simulink model "DemonstratorSimscape"  (R2020b)
settings: Solver=ode113  StartTime=0.0  StopTime=t_stop*0+20  FixedStep=1e-4
values from neighbouring files (symbols this model uses):
  brkD = 0    [main.m]
  brkI = 1e4    (= 10000)    [main.m]
  brkP = 1e5    (= 100000)    [main.m]
  d_drm = 0.5*d_drum    [main.m]
  d_shm = 0.4*d_sheave    [main.m]
  DeltaCable0 = 0    [main.m]
  Droop_scaling = 0    [main.m]
  eta_sh = 0.015    [main.m]
  filt_NUM = ones(1,200)*0.005    [main.m]
  g = 9.80665    [main.m]
  Iw = 0.5*(W.i + M.in*GB.r^2)    [main.m]
  Kp_mul = 0.3    [main.m]
  Lc0 = abs((T.ph-L.height-P.d-L.z0)*0.001)    [main.m]
  Ls1 = ((T.ph-0.5*W.pd)/1000)    [main.m]
  Ls2 = ((0.5*(T.s2+P.d)-2*P.d)/1000)    [main.m]
  M = 50e3    (= 50000)    [calcGrav.m]
  phi0_drm = -90    [main.m]
  phi0_shm = -90    [main.m]
  r_sheave = P.d*0.5    [main.m]
  s = tf('s')    [calcGrav.m]
  tau_brk = 0.001    [main.m]
  tau_em = 60e-3    (= 0.06)    [calcGrav.m]    (also in main.m)
  tau_m = tau_w/GB.r    [main.m]
  Tmax = 400e3    (= 400000)    [main.m]
  Tn_mul = 10    [main.m]
  x_drm = 0.7*r_drum    [main.m]
  x_shm = 0.7*r_sheave    [main.m]
  z0 = 0    [calcGrav.m]    (also in main.m = L.z0-P.d*0.5-P.d-P.d-L.height-T.h1-T.h2-32)
undefined symbols (not defined in the file or in its folder): C, CA, Controller_sampleTime, DiscIntNeverNeededParam, GB, L, P, Part, T, VFD_acceleration_model_factor, VFD_Adapt_factor_lower_p1458, VFD_Adapt_factor_upper_p1459, VFD_Curr_limit_var_p0641, VFD_Current_limit_p0640, VFD_Id_setp_total_r1624, VFD_Iq, VFD_Kp_n_basic_p1460, VFD_M, VFD_M_accel_T_smooth_p1517, VFD_M_lim_var_fixS_src_p1551, VFD_M_max_lower_p1521, VFD_M_max_lower_scal_p1525, VFD_M_max_up_mot_scal_p1524, VFD_M_max_upper_p1520, VFD_n_act_T_smooth_p1442, VFD_n_ctr_Kp_n_up_scal_p1461, VFD_n_ctr_Tn_n_up_sca_p1463, VFD_n_ctrl_adapt_Kp_lower_p1456, VFD_n_ctrl_adapt_Kp_upper_p1457, VFD_n_ctrl_Adpt_sig_Kp_p1455, VFD_n_ctrl_Kp_scal_p1466, VFD_n_ctrl_n_lower_p1464, VFD_n_ctrl_n_upper_p1465, VFD_n_ctrl_Tn_n_lower_p1462, VFD_n_limit_neg_p1086, VFD_n_limit_pos_p1083, VFD_n_limit_setp_p1063, VFD_n_max_p1082, VFD_n_set_filt_1_T_p1416, VFD_P_max_gen_p1531, VFD_P_max_mot_p1530, VFD_PU_I_outp_max_r0289, VFD_RFG_ramp_down_time_p1121, VFD_RFG_ramp_up_time_p1120, VFD_RFG_t_RD_scal_p1139, VFD_RFG_t_RU_scal_p1138, VSD, W, X, Y, Z
libraries: sm_lib x248, nesl_utility x128, simulink x49, pid_lib x4, cstblocks x2, simulink_extras x2
(part 10 of 10)

== system DemonstratorSimscape/Transmission System/Roof Pulley Set/Sheave_04/Pulley rught red2/tags ==
  Rigid Transform1 : sm_lib/Frames and Transforms/Rigid Transform  TranslationMethod=Cartesian  TranslationStandardOffset=0  TranslationLengthUnit=mm  TranslationStandardAxis=+Z  TranslationCartesianOffset=[x_shm*cosd(phi0+120), x_shm*sind(phi0+120), s*d_shm]  TranslationROffset=0  TranslationROffsetUnits=m  TranslationZOffset=0  TranslationZOffsetUnits=m  TranslationThetaOffset=0  TranslationThetaOffsetUnits=deg  RotationMethod=None  RotationAngleUnits=deg  RotationStandardAxis=+Z  RotationAngle=0.0  RotationArbitraryAxis=[0 0 1]  FollAlignAxisA=+X  BaseAlignAxisA=+Y  FollAlignAxisB=+Y  BaseAlignAxisB=+Z  RotationSequenceAxes=FollowerAxes  RotationSequence=XYX  RotationSequenceAngles=[0 0 0]  RotationSequenceAnglesUnits=deg  RotationMatrix=[1 0 0; 0 1 0; 0 0 1]
  Rigid Transform2 : sm_lib/Frames and Transforms/Rigid Transform  TranslationMethod=Cartesian  TranslationStandardOffset=0  TranslationLengthUnit=mm  TranslationStandardAxis=+Z  TranslationCartesianOffset=[x_shm*cosd(phi0+0), x_shm*sind(phi0+0), s*d_shm]  TranslationROffset=0  TranslationROffsetUnits=m  TranslationZOffset=0  TranslationZOffsetUnits=m  TranslationThetaOffset=0  TranslationThetaOffsetUnits=deg  RotationMethod=None  RotationAngleUnits=deg  RotationStandardAxis=+Z  RotationAngle=0.0  RotationArbitraryAxis=[0 0 1]  FollAlignAxisA=+X  BaseAlignAxisA=+Y  FollAlignAxisB=+Y  BaseAlignAxisB=+Z  RotationSequenceAxes=FollowerAxes  RotationSequence=XYX  RotationSequenceAngles=[0 0 0]  RotationSequenceAnglesUnits=deg  RotationMatrix=[1 0 0; 0 1 0; 0 0 1]
  Rigid Transform3 : sm_lib/Frames and Transforms/Rigid Transform  TranslationMethod=Cartesian  TranslationStandardOffset=0  TranslationLengthUnit=mm  TranslationStandardAxis=+Z  TranslationCartesianOffset=[x_shm*cosd(phi0-120), x_shm*sind(phi0-120), s*d_shm]  TranslationROffset=0  TranslationROffsetUnits=m  TranslationZOffset=0  TranslationZOffsetUnits=m  TranslationThetaOffset=0  TranslationThetaOffsetUnits=deg  RotationMethod=None  RotationAngleUnits=deg  RotationStandardAxis=+Z  RotationAngle=0.0  RotationArbitraryAxis=[0 0 1]  FollAlignAxisA=+X  BaseAlignAxisA=+Y  FollAlignAxisB=+Y  BaseAlignAxisB=+Z  RotationSequenceAxes=FollowerAxes  RotationSequence=XYX  RotationSequenceAngles=[0 0 0]  RotationSequenceAnglesUnits=deg  RotationMatrix=[1 0 0; 0 1 0; 0 0 1]
  tag1 : sm_lib/Body Elements/Cylindrical Solid  GraphicAmbientColor=[0.15 0.15 0.15 1.0]  BasedOnType=Density  CenterOfMass=[0 0 0]  CenterOfMassUnits=m  GraphicDiffuseColor=c_shm  CylinderLength=d_shm  CylinderLengthUnits=mm  CylinderRadius=r_shm  CylinderRadiusUnits=mm  Density=0  DensityUnits=kg/m^3  DoExposeReferenceFrame=on  GraphicEmissiveColor=[0.0 0.0 0.0 1.0]  ExportEntireGeometry=off  SerializedFrames=<Frames/>  MarkerShape=Frame  MarkerSize=10  GraphicType=FromGeometry  InertiaType=CalculateFromGeometry  Mass=0  MassUnits=kg  MomentsOfInertia=[1 1 1]  MomentsOfInertiaUnits=kg*m^2  GraphicOpacity=1.0  ProductsOfInertia=[0 0 0]  ProductsOfInertiaUnits=kg*m^2  GraphicShininess=10  GraphicSpecularColor=[0.8 0.8 0.8]  GraphicVisPropType=SimpleVisualProperties
  tag2 : sm_lib/Body Elements/Cylindrical Solid  GraphicAmbientColor=[0.15 0.15 0.15 1.0]  BasedOnType=Density  CenterOfMass=[0 0 0]  CenterOfMassUnits=m  GraphicDiffuseColor=c_shm  CylinderLength=d_shm  CylinderLengthUnits=mm  CylinderRadius=r_shm  CylinderRadiusUnits=mm  Density=0  DensityUnits=kg/m^3  DoExposeReferenceFrame=on  GraphicEmissiveColor=[0.0 0.0 0.0 1.0]  ExportEntireGeometry=off  SerializedFrames=<Frames/>  MarkerShape=Frame  MarkerSize=10  GraphicType=FromGeometry  InertiaType=CalculateFromGeometry  Mass=0  MassUnits=kg  MomentsOfInertia=[1 1 1]  MomentsOfInertiaUnits=kg*m^2  GraphicOpacity=1.0  ProductsOfInertia=[0 0 0]  ProductsOfInertiaUnits=kg*m^2  GraphicShininess=10  GraphicSpecularColor=[0.8 0.8 0.8]  GraphicVisPropType=SimpleVisualProperties
  tag3 : sm_lib/Body Elements/Cylindrical Solid  GraphicAmbientColor=[0.15 0.15 0.15 1.0]  BasedOnType=Density  CenterOfMass=[0 0 0]  CenterOfMassUnits=m  GraphicDiffuseColor=c_shm  CylinderLength=d_shm  CylinderLengthUnits=mm  CylinderRadius=r_shm  CylinderRadiusUnits=mm  Density=0  DensityUnits=kg/m^3  DoExposeReferenceFrame=on  GraphicEmissiveColor=[0.0 0.0 0.0 1.0]  ExportEntireGeometry=off  SerializedFrames=<Frames/>  MarkerShape=Frame  MarkerSize=10  GraphicType=FromGeometry  InertiaType=CalculateFromGeometry  Mass=0  MassUnits=kg  MomentsOfInertia=[1 1 1]  MomentsOfInertiaUnits=kg*m^2  GraphicOpacity=1.0  ProductsOfInertia=[0 0 0]  ProductsOfInertiaUnits=kg*m^2  GraphicShininess=10  GraphicSpecularColor=[0.8 0.8 0.8]  GraphicVisPropType=SimpleVisualProperties
  Conn1 : PMIOPort  Side=Left
  connections:
  tag2/RConn1 -- Rigid Transform1/RConn1
  Conn1/RConn1 -- Rigid Transform2/LConn1 -- Rigid Transform1/LConn1 -- Rigid Transform3/LConn1
  Rigid Transform2/RConn1 -- tag1/RConn1
  Rigid Transform3/RConn1 -- tag3/RConn1

== system DemonstratorSimscape/Transmission System/Roof Pulley Set/Sheave_06/Sheave6/tags ==
  Rigid Transform1 : sm_lib/Frames and Transforms/Rigid Transform  TranslationMethod=Cartesian  TranslationStandardOffset=0  TranslationLengthUnit=mm  TranslationStandardAxis=+Z  TranslationCartesianOffset=[x_shm*cosd(phi0+120), x_shm*sind(phi0+120), s*d_shm]  TranslationROffset=0  TranslationROffsetUnits=m  TranslationZOffset=0  TranslationZOffsetUnits=m  TranslationThetaOffset=0  TranslationThetaOffsetUnits=deg  RotationMethod=None  RotationAngleUnits=deg  RotationStandardAxis=+Z  RotationAngle=0.0  RotationArbitraryAxis=[0 0 1]  FollAlignAxisA=+X  BaseAlignAxisA=+Y  FollAlignAxisB=+Y  BaseAlignAxisB=+Z  RotationSequenceAxes=FollowerAxes  RotationSequence=XYX  RotationSequenceAngles=[0 0 0]  RotationSequenceAnglesUnits=deg  RotationMatrix=[1 0 0; 0 1 0; 0 0 1]
  Rigid Transform2 : sm_lib/Frames and Transforms/Rigid Transform  TranslationMethod=Cartesian  TranslationStandardOffset=0  TranslationLengthUnit=mm  TranslationStandardAxis=+Z  TranslationCartesianOffset=[x_shm*cosd(phi0+0), x_shm*sind(phi0+0), s*d_shm]  TranslationROffset=0  TranslationROffsetUnits=m  TranslationZOffset=0  TranslationZOffsetUnits=m  TranslationThetaOffset=0  TranslationThetaOffsetUnits=deg  RotationMethod=None  RotationAngleUnits=deg  RotationStandardAxis=+Z  RotationAngle=0.0  RotationArbitraryAxis=[0 0 1]  FollAlignAxisA=+X  BaseAlignAxisA=+Y  FollAlignAxisB=+Y  BaseAlignAxisB=+Z  RotationSequenceAxes=FollowerAxes  RotationSequence=XYX  RotationSequenceAngles=[0 0 0]  RotationSequenceAnglesUnits=deg  RotationMatrix=[1 0 0; 0 1 0; 0 0 1]
  Rigid Transform3 : sm_lib/Frames and Transforms/Rigid Transform  TranslationMethod=Cartesian  TranslationStandardOffset=0  TranslationLengthUnit=mm  TranslationStandardAxis=+Z  TranslationCartesianOffset=[x_shm*cosd(phi0-120), x_shm*sind(phi0-120), s*d_shm]  TranslationROffset=0  TranslationROffsetUnits=m  TranslationZOffset=0  TranslationZOffsetUnits=m  TranslationThetaOffset=0  TranslationThetaOffsetUnits=deg  RotationMethod=None  RotationAngleUnits=deg  RotationStandardAxis=+Z  RotationAngle=0.0  RotationArbitraryAxis=[0 0 1]  FollAlignAxisA=+X  BaseAlignAxisA=+Y  FollAlignAxisB=+Y  BaseAlignAxisB=+Z  RotationSequenceAxes=FollowerAxes  RotationSequence=XYX  RotationSequenceAngles=[0 0 0]  RotationSequenceAnglesUnits=deg  RotationMatrix=[1 0 0; 0 1 0; 0 0 1]
  tag1 : sm_lib/Body Elements/Cylindrical Solid  GraphicAmbientColor=[0.15 0.15 0.15 1.0]  BasedOnType=Density  CenterOfMass=[0 0 0]  CenterOfMassUnits=m  GraphicDiffuseColor=c_shm  CylinderLength=d_shm  CylinderLengthUnits=mm  CylinderRadius=r_shm  CylinderRadiusUnits=mm  Density=0  DensityUnits=kg/m^3  DoExposeReferenceFrame=on  GraphicEmissiveColor=[0.0 0.0 0.0 1.0]  ExportEntireGeometry=off  SerializedFrames=<Frames/>  MarkerShape=Frame  MarkerSize=10  GraphicType=FromGeometry  InertiaType=CalculateFromGeometry  Mass=0  MassUnits=kg  MomentsOfInertia=[1 1 1]  MomentsOfInertiaUnits=kg*m^2  GraphicOpacity=1.0  ProductsOfInertia=[0 0 0]  ProductsOfInertiaUnits=kg*m^2  GraphicShininess=10  GraphicSpecularColor=[0.8 0.8 0.8]  GraphicVisPropType=SimpleVisualProperties
  tag2 : sm_lib/Body Elements/Cylindrical Solid  GraphicAmbientColor=[0.15 0.15 0.15 1.0]  BasedOnType=Density  CenterOfMass=[0 0 0]  CenterOfMassUnits=m  GraphicDiffuseColor=c_shm  CylinderLength=d_shm  CylinderLengthUnits=mm  CylinderRadius=r_shm  CylinderRadiusUnits=mm  Density=0  DensityUnits=kg/m^3  DoExposeReferenceFrame=on  GraphicEmissiveColor=[0.0 0.0 0.0 1.0]  ExportEntireGeometry=off  SerializedFrames=<Frames/>  MarkerShape=Frame  MarkerSize=10  GraphicType=FromGeometry  InertiaType=CalculateFromGeometry  Mass=0  MassUnits=kg  MomentsOfInertia=[1 1 1]  MomentsOfInertiaUnits=kg*m^2  GraphicOpacity=1.0  ProductsOfInertia=[0 0 0]  ProductsOfInertiaUnits=kg*m^2  GraphicShininess=10  GraphicSpecularColor=[0.8 0.8 0.8]  GraphicVisPropType=SimpleVisualProperties
  tag3 : sm_lib/Body Elements/Cylindrical Solid  GraphicAmbientColor=[0.15 0.15 0.15 1.0]  BasedOnType=Density  CenterOfMass=[0 0 0]  CenterOfMassUnits=m  GraphicDiffuseColor=c_shm  CylinderLength=d_shm  CylinderLengthUnits=mm  CylinderRadius=r_shm  CylinderRadiusUnits=mm  Density=0  DensityUnits=kg/m^3  DoExposeReferenceFrame=on  GraphicEmissiveColor=[0.0 0.0 0.0 1.0]  ExportEntireGeometry=off  SerializedFrames=<Frames/>  MarkerShape=Frame  MarkerSize=10  GraphicType=FromGeometry  InertiaType=CalculateFromGeometry  Mass=0  MassUnits=kg  MomentsOfInertia=[1 1 1]  MomentsOfInertiaUnits=kg*m^2  GraphicOpacity=1.0  ProductsOfInertia=[0 0 0]  ProductsOfInertiaUnits=kg*m^2  GraphicShininess=10  GraphicSpecularColor=[0.8 0.8 0.8]  GraphicVisPropType=SimpleVisualProperties
  Conn1 : PMIOPort  Side=Left
  connections:
  tag2/RConn1 -- Rigid Transform1/RConn1
  Conn1/RConn1 -- Rigid Transform2/LConn1 -- Rigid Transform1/LConn1 -- Rigid Transform3/LConn1
  Rigid Transform2/RConn1 -- tag1/RConn1
  Rigid Transform3/RConn1 -- tag3/RConn1

== system DemonstratorSimscape/Transmission System/Roof Pulley Set/Sheave_07/Sheave7/tags ==
  Rigid Transform1 : sm_lib/Frames and Transforms/Rigid Transform  TranslationMethod=Cartesian  TranslationStandardOffset=0  TranslationLengthUnit=mm  TranslationStandardAxis=+Z  TranslationCartesianOffset=[x_shm*cosd(phi0+120), x_shm*sind(phi0+120), s*d_shm]  TranslationROffset=0  TranslationROffsetUnits=m  TranslationZOffset=0  TranslationZOffsetUnits=m  TranslationThetaOffset=0  TranslationThetaOffsetUnits=deg  RotationMethod=None  RotationAngleUnits=deg  RotationStandardAxis=+Z  RotationAngle=0.0  RotationArbitraryAxis=[0 0 1]  FollAlignAxisA=+X  BaseAlignAxisA=+Y  FollAlignAxisB=+Y  BaseAlignAxisB=+Z  RotationSequenceAxes=FollowerAxes  RotationSequence=XYX  RotationSequenceAngles=[0 0 0]  RotationSequenceAnglesUnits=deg  RotationMatrix=[1 0 0; 0 1 0; 0 0 1]
  Rigid Transform2 : sm_lib/Frames and Transforms/Rigid Transform  TranslationMethod=Cartesian  TranslationStandardOffset=0  TranslationLengthUnit=mm  TranslationStandardAxis=+Z  TranslationCartesianOffset=[x_shm*cosd(phi0+0), x_shm*sind(phi0+0), s*d_shm]  TranslationROffset=0  TranslationROffsetUnits=m  TranslationZOffset=0  TranslationZOffsetUnits=m  TranslationThetaOffset=0  TranslationThetaOffsetUnits=deg  RotationMethod=None  RotationAngleUnits=deg  RotationStandardAxis=+Z  RotationAngle=0.0  RotationArbitraryAxis=[0 0 1]  FollAlignAxisA=+X  BaseAlignAxisA=+Y  FollAlignAxisB=+Y  BaseAlignAxisB=+Z  RotationSequenceAxes=FollowerAxes  RotationSequence=XYX  RotationSequenceAngles=[0 0 0]  RotationSequenceAnglesUnits=deg  RotationMatrix=[1 0 0; 0 1 0; 0 0 1]
  Rigid Transform3 : sm_lib/Frames and Transforms/Rigid Transform  TranslationMethod=Cartesian  TranslationStandardOffset=0  TranslationLengthUnit=mm  TranslationStandardAxis=+Z  TranslationCartesianOffset=[x_shm*cosd(phi0-120), x_shm*sind(phi0-120), s*d_shm]  TranslationROffset=0  TranslationROffsetUnits=m  TranslationZOffset=0  TranslationZOffsetUnits=m  TranslationThetaOffset=0  TranslationThetaOffsetUnits=deg  RotationMethod=None  RotationAngleUnits=deg  RotationStandardAxis=+Z  RotationAngle=0.0  RotationArbitraryAxis=[0 0 1]  FollAlignAxisA=+X  BaseAlignAxisA=+Y  FollAlignAxisB=+Y  BaseAlignAxisB=+Z  RotationSequenceAxes=FollowerAxes  RotationSequence=XYX  RotationSequenceAngles=[0 0 0]  RotationSequenceAnglesUnits=deg  RotationMatrix=[1 0 0; 0 1 0; 0 0 1]
  tag1 : sm_lib/Body Elements/Cylindrical Solid  GraphicAmbientColor=[0.15 0.15 0.15 1.0]  BasedOnType=Density  CenterOfMass=[0 0 0]  CenterOfMassUnits=m  GraphicDiffuseColor=c_shm  CylinderLength=d_shm  CylinderLengthUnits=mm  CylinderRadius=r_shm  CylinderRadiusUnits=mm  Density=0  DensityUnits=kg/m^3  DoExposeReferenceFrame=on  GraphicEmissiveColor=[0.0 0.0 0.0 1.0]  ExportEntireGeometry=off  SerializedFrames=<Frames/>  MarkerShape=Frame  MarkerSize=10  GraphicType=FromGeometry  InertiaType=CalculateFromGeometry  Mass=0  MassUnits=kg  MomentsOfInertia=[1 1 1]  MomentsOfInertiaUnits=kg*m^2  GraphicOpacity=1.0  ProductsOfInertia=[0 0 0]  ProductsOfInertiaUnits=kg*m^2  GraphicShininess=10  GraphicSpecularColor=[0.8 0.8 0.8]  GraphicVisPropType=SimpleVisualProperties
  tag2 : sm_lib/Body Elements/Cylindrical Solid  GraphicAmbientColor=[0.15 0.15 0.15 1.0]  BasedOnType=Density  CenterOfMass=[0 0 0]  CenterOfMassUnits=m  GraphicDiffuseColor=c_shm  CylinderLength=d_shm  CylinderLengthUnits=mm  CylinderRadius=r_shm  CylinderRadiusUnits=mm  Density=0  DensityUnits=kg/m^3  DoExposeReferenceFrame=on  GraphicEmissiveColor=[0.0 0.0 0.0 1.0]  ExportEntireGeometry=off  SerializedFrames=<Frames/>  MarkerShape=Frame  MarkerSize=10  GraphicType=FromGeometry  InertiaType=CalculateFromGeometry  Mass=0  MassUnits=kg  MomentsOfInertia=[1 1 1]  MomentsOfInertiaUnits=kg*m^2  GraphicOpacity=1.0  ProductsOfInertia=[0 0 0]  ProductsOfInertiaUnits=kg*m^2  GraphicShininess=10  GraphicSpecularColor=[0.8 0.8 0.8]  GraphicVisPropType=SimpleVisualProperties
  tag3 : sm_lib/Body Elements/Cylindrical Solid  GraphicAmbientColor=[0.15 0.15 0.15 1.0]  BasedOnType=Density  CenterOfMass=[0 0 0]  CenterOfMassUnits=m  GraphicDiffuseColor=c_shm  CylinderLength=d_shm  CylinderLengthUnits=mm  CylinderRadius=r_shm  CylinderRadiusUnits=mm  Density=0  DensityUnits=kg/m^3  DoExposeReferenceFrame=on  GraphicEmissiveColor=[0.0 0.0 0.0 1.0]  ExportEntireGeometry=off  SerializedFrames=<Frames/>  MarkerShape=Frame  MarkerSize=10  GraphicType=FromGeometry  InertiaType=CalculateFromGeometry  Mass=0  MassUnits=kg  MomentsOfInertia=[1 1 1]  MomentsOfInertiaUnits=kg*m^2  GraphicOpacity=1.0  ProductsOfInertia=[0 0 0]  ProductsOfInertiaUnits=kg*m^2  GraphicShininess=10  GraphicSpecularColor=[0.8 0.8 0.8]  GraphicVisPropType=SimpleVisualProperties
  Conn1 : PMIOPort  Side=Left
  connections:
  tag2/RConn1 -- Rigid Transform1/RConn1
  Conn1/RConn1 -- Rigid Transform2/LConn1 -- Rigid Transform1/LConn1 -- Rigid Transform3/LConn1
  Rigid Transform2/RConn1 -- tag1/RConn1
  Rigid Transform3/RConn1 -- tag3/RConn1

== system DemonstratorSimscape/EM System/Drives/PLC and Drive Logic Rev3/VFD Control1/[6020] Speed control and generation of the torque limits /1st order LPF ==
  Signal : Inport
  Time Constant : Inport  Port=2
  Add1 : Sum
  Add3 : Sum
  Add4 : Sum  Inputs=+-
  Constant1 : Constant  Value=Controller_sampleTime
  Divide : Product  Inputs=*/
  Memory1 : Memory  InitialCondition=Yo  InheritSampleTime=on
  Product1 : Product  RndMeth=Zero
  Signal Out : Outport  VectorParamsAs1DForOutWhenUnconnected=off
  wires:
  Signal/1 -> Add4/1
  Constant1/1 -> Divide/1, Add1/1
  Time Constant/1 -> Add1/2
  Add4/1 -> Product1/2
  Memory1/1 -> Add3/1, Add4/2
  Product1/1 -> Add3/2
  Add3/1 -> Signal Out/1, Memory1/1
  Divide/1 -> Product1/1
  Add1/1 -> Divide/2

== system DemonstratorSimscape/EM System/Drives/PLC and Drive Logic Rev3/VFD Control1/[6020] Speed control and generation of the torque limits /1st order LPF1 ==
  Signal : Inport
  Time Constant : Inport  Port=2
  Add1 : Sum
  Add3 : Sum
  Add4 : Sum  Inputs=+-
  Constant1 : Constant  Value=Controller_sampleTime
  Divide : Product  Inputs=*/
  Memory1 : Memory  InitialCondition=Yo  InheritSampleTime=on
  Product1 : Product  RndMeth=Zero
  Signal Out : Outport  VectorParamsAs1DForOutWhenUnconnected=off
  wires:
  Signal/1 -> Add4/1
  Constant1/1 -> Divide/1, Add1/1
  Time Constant/1 -> Add1/2
  Add4/1 -> Product1/2
  Memory1/1 -> Add3/1, Add4/2
  Product1/1 -> Add3/2
  Add3/1 -> Signal Out/1, Memory1/1
  Divide/1 -> Product1/1
  Add1/1 -> Divide/2

== system DemonstratorSimscape/EM System/Drives/PLC and Drive Logic Rev3/VFD Control1/[6020] Speed control and generation of the torque limits /1st order LPF2 ==
  Signal : Inport
  Time Constant : Inport  Port=2
  Add1 : Sum
  Add3 : Sum
  Add4 : Sum  Inputs=+-
  Constant1 : Constant  Value=Controller_sampleTime
  Divide : Product  Inputs=*/
  Memory1 : Memory  InitialCondition=Yo  InheritSampleTime=on
  Product1 : Product  RndMeth=Zero
  Signal Out : Outport  VectorParamsAs1DForOutWhenUnconnected=off
  wires:
  Add1/1 -> Divide/2
  Divide/1 -> Product1/1
  Add3/1 -> Memory1/1, Signal Out/1
  Product1/1 -> Add3/2
  Memory1/1 -> Add4/2, Add3/1
  Add4/1 -> Product1/2
  Time Constant/1 -> Add1/2
  Constant1/1 -> Add1/1, Divide/1
  Signal/1 -> Add4/1

== system DemonstratorSimscape/EM System/Drives/PLC and Drive Logic Rev3/VFD Control1/[6020] Speed control and generation of the torque limits /1st order LPF3 ==
  Signal : Inport
  Time Constant : Inport  Port=2
  Add1 : Sum
  Add3 : Sum
  Add4 : Sum  Inputs=+-
  Constant1 : Constant  Value=Controller_sampleTime
  Divide : Product  Inputs=*/
  Memory1 : Memory  InitialCondition=Yo  InheritSampleTime=on
  Product1 : Product  RndMeth=Zero
  Signal Out : Outport  VectorParamsAs1DForOutWhenUnconnected=off
  wires:
  Signal/1 -> Add4/1
  Constant1/1 -> Divide/1, Add1/1
  Time Constant/1 -> Add1/2
  Add4/1 -> Product1/2
  Memory1/1 -> Add3/1, Add4/2
  Product1/1 -> Add3/2
  Add3/1 -> Signal Out/1, Memory1/1
  Divide/1 -> Product1/1
  Add1/1 -> Divide/2

== system DemonstratorSimscape/EM System/Drives/PLC and Drive Logic Rev3/VFD Control1/[6020] Speed control and generation of the torque limits /[6050] Kp_n-//Tn_n adaptation NOTE: THE PARAMETERS USED CAUSE FIXED GAINS ==
  Measured_RPM_r0063 : Inport
  Abs : Abs
  Abs1 : Abs
  Adaptation factor lower : Constant  Value=VFD_Adapt_factor_lower_p1458
  "Adaptation factor upper " : Constant  Value=VFD_Adapt_factor_upper_p1459
  Free Kp_n adaptation : simulink/Lookup Tables/Lookup Table Dynamic  LookUpMeth=Interpolation-Use End Values  OutDataType=fixdt('double')  OutScaling=[]  OutputDataTypeScalingMode=Specify via dialog  OutDataTypeStr=double  DoSatur=off
  Mux{,1..4} (5 alike) : Mux  Inputs=2
  Product{1,6..8} (4 alike) : Product  Inputs=**
  Speed controller Kp adaptation speed upper scaling : Constant  Value=VFD_n_ctr_Kp_n_up_scal_p1461
  Speed controller P gain adaptation lower starting point : Constant  Value=VFD_n_ctrl_adapt_Kp_lower_p1456
  "Speed controller P gain adaptation signal " : Constant  Value=VFD_n_ctrl_Adpt_sig_Kp_p1455
  Speed controller P gain adaptation speed lower : Constant  Value=VFD_Kp_n_basic_p1460
  Speed controller P gain adaptation upper starting point : Constant  Value=VFD_n_ctrl_adapt_Kp_upper_p1457
  Speed controller P-gain scaling : Constant  Value=VFD_n_ctrl_Kp_scal_p1466
  Speed controller Tn adaptation speed upper scaling : Constant  Value=VFD_n_ctr_Tn_n_up_sca_p1463
  "Speed controller adaptation speed lower " : Constant  Value=VFD_n_ctrl_n_lower_p1464
  Speed controller adaptation speed upper : Constant  Value=VFD_n_ctrl_n_upper_p1465
  Speed controller integral time adaptation speed lower : Constant  Value=VFD_n_ctrl_Tn_n_lower_p1462
  Speed-dependent Kp_n adaptation : simulink/Lookup Tables/Lookup Table Dynamic  LookUpMeth=Interpolation-Use End Values  OutDataType=fixdt('double')  OutScaling=[]  OutputDataTypeScalingMode=Specify via dialog  OutDataTypeStr=double  DoSatur=off
  Speed-dependent Tn_n adaptation : simulink/Lookup Tables/Lookup Table Dynamic  LookUpMeth=Interpolation-Use End Values  OutDataType=fixdt('double')  OutScaling=[]  OutputDataTypeScalingMode=Specify via dialog  OutDataTypeStr=double  DoSatur=off
  Kp_n_adapt : Outport
  Tn_n_adapt : Outport  Port=2
  wires:
  Product1/1 -> Mux/2
  Abs/1 -> Speed-dependent Kp_n adaptation/1, Speed-dependent Tn_n adaptation/1
  Abs1/1 -> Product7/2
  Adaptation factor lower/1 -> Mux3/1
  "Speed controller adaptation speed lower "/1 -> Mux2/1
  "Speed controller P gain adaptation signal "/1 -> Free Kp_n adaptation/1
  Speed controller integral time adaptation speed lower/1 -> Mux1/1, Product6/1
  Speed-dependent Tn_n adaptation/1 -> Tn_n_adapt/1  "Tn"
  Speed controller P gain adaptation speed lower/1 -> Product1/1, Mux/1
  Speed-dependent Kp_n adaptation/1 -> Product8/2  "Kp"
  Speed controller Tn adaptation speed upper scaling/1 -> Product6/2
  Mux1/1 -> Speed-dependent Tn_n adaptation/3
  Mux2/1 -> Speed-dependent Kp_n adaptation/2, Speed-dependent Tn_n adaptation/2
  Product7/1 -> Product8/1
  Product6/1 -> Mux1/2
  Speed controller adaptation speed upper/1 -> Mux2/2
  Speed controller P-gain scaling/1 -> Abs1/1
  Speed controller Kp adaptation speed upper scaling/1 -> Product1/2
  Measured_RPM_r0063/1 -> Abs/1
  Free Kp_n adaptation/1 -> Product7/1  "Kp"
  Mux/1 -> Speed-dependent Kp_n adaptation/3
  Speed controller P gain adaptation lower starting point/1 -> Mux4/1
  Speed controller P gain adaptation upper starting point/1 -> Mux4/2
  Mux3/1 -> Free Kp_n adaptation/3
  "Adaptation factor upper "/1 -> Mux3/2
  Mux4/1 -> Free Kp_n adaptation/2
  Product8/1 -> Kp_n_adapt/1

== system DemonstratorSimscape/EM System/Drives/PLC and Drive Logic Rev3/VFD Control2/[6020] Speed control and generation of the torque limits /1st order LPF ==
  Signal : Inport
  Time Constant : Inport  Port=2
  Add1 : Sum
  Add3 : Sum
  Add4 : Sum  Inputs=+-
  Constant1 : Constant  Value=Controller_sampleTime
  Divide : Product  Inputs=*/
  Memory1 : Memory  InitialCondition=Yo  InheritSampleTime=on
  Product1 : Product  RndMeth=Zero
  Signal Out : Outport  VectorParamsAs1DForOutWhenUnconnected=off
  wires:
  Signal/1 -> Add4/1
  Constant1/1 -> Divide/1, Add1/1
  Time Constant/1 -> Add1/2
  Add4/1 -> Product1/2
  Memory1/1 -> Add3/1, Add4/2
  Product1/1 -> Add3/2
  Add3/1 -> Signal Out/1, Memory1/1
  Divide/1 -> Product1/1
  Add1/1 -> Divide/2

== system DemonstratorSimscape/EM System/Drives/PLC and Drive Logic Rev3/VFD Control2/[6020] Speed control and generation of the torque limits /1st order LPF1 ==
  Signal : Inport
  Time Constant : Inport  Port=2
  Add1 : Sum
  Add3 : Sum
  Add4 : Sum  Inputs=+-
  Constant1 : Constant  Value=Controller_sampleTime
  Divide : Product  Inputs=*/
  Memory1 : Memory  InitialCondition=Yo  InheritSampleTime=on
  Product1 : Product  RndMeth=Zero
  Signal Out : Outport  VectorParamsAs1DForOutWhenUnconnected=off
  wires:
  Signal/1 -> Add4/1
  Constant1/1 -> Divide/1, Add1/1
  Time Constant/1 -> Add1/2
  Add4/1 -> Product1/2
  Memory1/1 -> Add3/1, Add4/2
  Product1/1 -> Add3/2
  Add3/1 -> Signal Out/1, Memory1/1
  Divide/1 -> Product1/1
  Add1/1 -> Divide/2

== system DemonstratorSimscape/EM System/Drives/PLC and Drive Logic Rev3/VFD Control2/[6020] Speed control and generation of the torque limits /1st order LPF2 ==
  Signal : Inport
  Time Constant : Inport  Port=2
  Add1 : Sum
  Add3 : Sum
  Add4 : Sum  Inputs=+-
  Constant1 : Constant  Value=Controller_sampleTime
  Divide : Product  Inputs=*/
  Memory1 : Memory  InitialCondition=Yo  InheritSampleTime=on
  Product1 : Product  RndMeth=Zero
  Signal Out : Outport  VectorParamsAs1DForOutWhenUnconnected=off
  wires:
  Add1/1 -> Divide/2
  Divide/1 -> Product1/1
  Add3/1 -> Memory1/1, Signal Out/1
  Product1/1 -> Add3/2
  Memory1/1 -> Add4/2, Add3/1
  Add4/1 -> Product1/2
  Time Constant/1 -> Add1/2
  Constant1/1 -> Add1/1, Divide/1
  Signal/1 -> Add4/1

== system DemonstratorSimscape/EM System/Drives/PLC and Drive Logic Rev3/VFD Control2/[6020] Speed control and generation of the torque limits /1st order LPF3 ==
  Signal : Inport
  Time Constant : Inport  Port=2
  Add1 : Sum
  Add3 : Sum
  Add4 : Sum  Inputs=+-
  Constant1 : Constant  Value=Controller_sampleTime
  Divide : Product  Inputs=*/
  Memory1 : Memory  InitialCondition=Yo  InheritSampleTime=on
  Product1 : Product  RndMeth=Zero
  Signal Out : Outport  VectorParamsAs1DForOutWhenUnconnected=off
  wires:
  Signal/1 -> Add4/1
  Constant1/1 -> Divide/1, Add1/1
  Time Constant/1 -> Add1/2
  Add4/1 -> Product1/2
  Memory1/1 -> Add3/1, Add4/2
  Product1/1 -> Add3/2
  Add3/1 -> Signal Out/1, Memory1/1
  Divide/1 -> Product1/1
  Add1/1 -> Divide/2

== system DemonstratorSimscape/EM System/Drives/PLC and Drive Logic Rev3/VFD Control2/[6020] Speed control and generation of the torque limits /[6050] Kp_n-//Tn_n adaptation NOTE: THE PARAMETERS USED CAUSE FIXED GAINS ==
  Measured_RPM_r0063 : Inport
  Abs : Abs
  Abs1 : Abs
  Adaptation factor lower : Constant  Value=VFD_Adapt_factor_lower_p1458
  "Adaptation factor upper " : Constant  Value=VFD_Adapt_factor_upper_p1459
  Free Kp_n adaptation : simulink/Lookup Tables/Lookup Table Dynamic  LookUpMeth=Interpolation-Use End Values  OutDataType=fixdt('double')  OutScaling=[]  OutputDataTypeScalingMode=Specify via dialog  OutDataTypeStr=double  DoSatur=off
  Mux{,1..4} (5 alike) : Mux  Inputs=2
  Product{1,6..8} (4 alike) : Product  Inputs=**
  Speed controller Kp adaptation speed upper scaling : Constant  Value=VFD_n_ctr_Kp_n_up_scal_p1461
  Speed controller P gain adaptation lower starting point : Constant  Value=VFD_n_ctrl_adapt_Kp_lower_p1456
  "Speed controller P gain adaptation signal " : Constant  Value=VFD_n_ctrl_Adpt_sig_Kp_p1455
  Speed controller P gain adaptation speed lower : Constant  Value=VFD_Kp_n_basic_p1460
  Speed controller P gain adaptation upper starting point : Constant  Value=VFD_n_ctrl_adapt_Kp_upper_p1457
  Speed controller P-gain scaling : Constant  Value=VFD_n_ctrl_Kp_scal_p1466
  Speed controller Tn adaptation speed upper scaling : Constant  Value=VFD_n_ctr_Tn_n_up_sca_p1463
  "Speed controller adaptation speed lower " : Constant  Value=VFD_n_ctrl_n_lower_p1464
  Speed controller adaptation speed upper : Constant  Value=VFD_n_ctrl_n_upper_p1465
  Speed controller integral time adaptation speed lower : Constant  Value=VFD_n_ctrl_Tn_n_lower_p1462
  Speed-dependent Kp_n adaptation : simulink/Lookup Tables/Lookup Table Dynamic  LookUpMeth=Interpolation-Use End Values  OutDataType=fixdt('double')  OutScaling=[]  OutputDataTypeScalingMode=Specify via dialog  OutDataTypeStr=double  DoSatur=off
  Speed-dependent Tn_n adaptation : simulink/Lookup Tables/Lookup Table Dynamic  LookUpMeth=Interpolation-Use End Values  OutDataType=fixdt('double')  OutScaling=[]  OutputDataTypeScalingMode=Specify via dialog  OutDataTypeStr=double  DoSatur=off
  Kp_n_adapt : Outport
  Tn_n_adapt : Outport  Port=2
  wires:
  Product1/1 -> Mux/2
  Abs/1 -> Speed-dependent Kp_n adaptation/1, Speed-dependent Tn_n adaptation/1
  Abs1/1 -> Product7/2
  Adaptation factor lower/1 -> Mux3/1
  "Speed controller adaptation speed lower "/1 -> Mux2/1
  "Speed controller P gain adaptation signal "/1 -> Free Kp_n adaptation/1
  Speed controller integral time adaptation speed lower/1 -> Mux1/1, Product6/1
  Speed-dependent Tn_n adaptation/1 -> Tn_n_adapt/1  "Tn"
  Speed controller P gain adaptation speed lower/1 -> Product1/1, Mux/1
  Speed-dependent Kp_n adaptation/1 -> Product8/2  "Kp"
  Speed controller Tn adaptation speed upper scaling/1 -> Product6/2
  Mux1/1 -> Speed-dependent Tn_n adaptation/3
  Mux2/1 -> Speed-dependent Kp_n adaptation/2, Speed-dependent Tn_n adaptation/2
  Product7/1 -> Product8/1
  Product6/1 -> Mux1/2
  Speed controller adaptation speed upper/1 -> Mux2/2
  Speed controller P-gain scaling/1 -> Abs1/1
  Speed controller Kp adaptation speed upper scaling/1 -> Product1/2
  Measured_RPM_r0063/1 -> Abs/1
  Free Kp_n adaptation/1 -> Product7/1  "Kp"
  Mux/1 -> Speed-dependent Kp_n adaptation/3
  Speed controller P gain adaptation lower starting point/1 -> Mux4/1
  Speed controller P gain adaptation upper starting point/1 -> Mux4/2
  Mux3/1 -> Free Kp_n adaptation/3
  "Adaptation factor upper "/1 -> Mux3/2
  Mux4/1 -> Free Kp_n adaptation/2
  Product8/1 -> Kp_n_adapt/1

== system DemonstratorSimscape/Transmission System/Anchor and Load/Load/DOUBLE/Planar Load1/PS>Sim2 ==
  a (m/s^2) : nesl_utility/PS-Simulink Converter  PhysicalDomain=network_engine_domain  SubClassName=ps_output  LeftPortType=input  RightPortType=output  PseudoPeriodic=off  Frequencies=[]  Unit=m/s^2  AffineConversion=off
  f (N) : nesl_utility/PS-Simulink Converter  PhysicalDomain=network_engine_domain  SubClassName=ps_output  LeftPortType=input  RightPortType=output  PseudoPeriodic=off  Frequencies=[]  Unit=N  AffineConversion=off
  fc (N) : nesl_utility/PS-Simulink Converter  PhysicalDomain=network_engine_domain  SubClassName=ps_output  LeftPortType=input  RightPortType=output  PseudoPeriodic=off  Frequencies=[]  Unit=N  AffineConversion=off
  ft (N) : nesl_utility/PS-Simulink Converter  PhysicalDomain=network_engine_domain  SubClassName=ps_output  LeftPortType=input  RightPortType=output  PseudoPeriodic=off  Frequencies=[]  Unit=N  AffineConversion=off
  p (m) : nesl_utility/PS-Simulink Converter  PhysicalDomain=network_engine_domain  SubClassName=ps_output  LeftPortType=input  RightPortType=output  PseudoPeriodic=off  Frequencies=[]  Unit=m  AffineConversion=off
  tc (Nm) : nesl_utility/PS-Simulink Converter  PhysicalDomain=network_engine_domain  SubClassName=ps_output  LeftPortType=input  RightPortType=output  PseudoPeriodic=off  Frequencies=[]  Unit=N*m  AffineConversion=off
  tt (Nm) : nesl_utility/PS-Simulink Converter  PhysicalDomain=network_engine_domain  SubClassName=ps_output  LeftPortType=input  RightPortType=output  PseudoPeriodic=off  Frequencies=[]  Unit=N*m  AffineConversion=off
  v (m/s) : nesl_utility/PS-Simulink Converter  PhysicalDomain=network_engine_domain  SubClassName=ps_output  LeftPortType=input  RightPortType=output  PseudoPeriodic=off  Frequencies=[]  Unit=m/s  AffineConversion=off
  q : PMIOPort  Side=Left
  Conn2 : PMIOPort  Port=2  Side=Left
  Conn3 : PMIOPort  Port=3  Side=Left
  Conn4 : PMIOPort  Port=4  Side=Left
  Conn5 : PMIOPort  Port=5  Side=Left
  Conn6 : PMIOPort  Port=6  Side=Left
  Conn7 : PMIOPort  Port=7  Side=Left
  Conn8 : PMIOPort  Port=8  Side=Left
  Out1 : Outport  VectorParamsAs1DForOutWhenUnconnected=off
  Out2 : Outport  Port=2  VectorParamsAs1DForOutWhenUnconnected=off
  Out3 : Outport  Port=3  VectorParamsAs1DForOutWhenUnconnected=off
  Out4 : Outport  Port=4  VectorParamsAs1DForOutWhenUnconnected=off
  Out5 : Outport  Port=5  VectorParamsAs1DForOutWhenUnconnected=off
  Out6 : Outport  Port=6  VectorParamsAs1DForOutWhenUnconnected=off
  Out7 : Outport  Port=7  VectorParamsAs1DForOutWhenUnconnected=off
  Out8 : Outport  Port=8  VectorParamsAs1DForOutWhenUnconnected=off
  wires:
  p (m)/1 -> Out1/1
  v (m/s)/1 -> Out2/1
  a (m/s^2)/1 -> Out3/1
  f (N)/1 -> Out4/1
  fc (N)/1 -> Out5/1
  tc (Nm)/1 -> Out6/1
  ft (N)/1 -> Out7/1
  tt (Nm)/1 -> Out8/1
  connections:
  q/RConn1 -- p (m)/LConn1
  Conn2/RConn1 -- v (m/s)/LConn1
  Conn3/RConn1 -- a (m/s^2)/LConn1
  Conn4/RConn1 -- f (N)/LConn1
  fc (N)/LConn1 -- Conn5/RConn1
  Conn6/RConn1 -- tc (Nm)/LConn1
  ft (N)/LConn1 -- Conn7/RConn1
  Conn8/RConn1 -- tt (Nm)/LConn1

== system DemonstratorSimscape/Transmission System/Anchor and Load/Load/DOUBLE/Planar Load2/PS>Sim2 ==
  a (m/s^2) : nesl_utility/PS-Simulink Converter  PhysicalDomain=network_engine_domain  SubClassName=ps_output  LeftPortType=input  RightPortType=output  PseudoPeriodic=off  Frequencies=[]  Unit=m/s^2  AffineConversion=off
  f (N) : nesl_utility/PS-Simulink Converter  PhysicalDomain=network_engine_domain  SubClassName=ps_output  LeftPortType=input  RightPortType=output  PseudoPeriodic=off  Frequencies=[]  Unit=N  AffineConversion=off
  fc (N) : nesl_utility/PS-Simulink Converter  PhysicalDomain=network_engine_domain  SubClassName=ps_output  LeftPortType=input  RightPortType=output  PseudoPeriodic=off  Frequencies=[]  Unit=N  AffineConversion=off
  ft (N) : nesl_utility/PS-Simulink Converter  PhysicalDomain=network_engine_domain  SubClassName=ps_output  LeftPortType=input  RightPortType=output  PseudoPeriodic=off  Frequencies=[]  Unit=N  AffineConversion=off
  p (m) : nesl_utility/PS-Simulink Converter  PhysicalDomain=network_engine_domain  SubClassName=ps_output  LeftPortType=input  RightPortType=output  PseudoPeriodic=off  Frequencies=[]  Unit=m  AffineConversion=off
  tc (Nm) : nesl_utility/PS-Simulink Converter  PhysicalDomain=network_engine_domain  SubClassName=ps_output  LeftPortType=input  RightPortType=output  PseudoPeriodic=off  Frequencies=[]  Unit=N*m  AffineConversion=off
  tt (Nm) : nesl_utility/PS-Simulink Converter  PhysicalDomain=network_engine_domain  SubClassName=ps_output  LeftPortType=input  RightPortType=output  PseudoPeriodic=off  Frequencies=[]  Unit=N*m  AffineConversion=off
  v (m/s) : nesl_utility/PS-Simulink Converter  PhysicalDomain=network_engine_domain  SubClassName=ps_output  LeftPortType=input  RightPortType=output  PseudoPeriodic=off  Frequencies=[]  Unit=m/s  AffineConversion=off
  q : PMIOPort  Side=Left
  Conn2 : PMIOPort  Port=2  Side=Left
  Conn3 : PMIOPort  Port=3  Side=Left
  Conn4 : PMIOPort  Port=4  Side=Left
  Conn5 : PMIOPort  Port=5  Side=Left
  Conn6 : PMIOPort  Port=6  Side=Left
  Conn7 : PMIOPort  Port=7  Side=Left
  Conn8 : PMIOPort  Port=8  Side=Left
  Out1 : Outport  VectorParamsAs1DForOutWhenUnconnected=off
  Out2 : Outport  Port=2  VectorParamsAs1DForOutWhenUnconnected=off
  Out3 : Outport  Port=3  VectorParamsAs1DForOutWhenUnconnected=off
  Out4 : Outport  Port=4  VectorParamsAs1DForOutWhenUnconnected=off
  Out5 : Outport  Port=5  VectorParamsAs1DForOutWhenUnconnected=off
  Out6 : Outport  Port=6  VectorParamsAs1DForOutWhenUnconnected=off
  Out7 : Outport  Port=7  VectorParamsAs1DForOutWhenUnconnected=off
  Out8 : Outport  Port=8  VectorParamsAs1DForOutWhenUnconnected=off
  wires:
  p (m)/1 -> Out1/1
  v (m/s)/1 -> Out2/1
  a (m/s^2)/1 -> Out3/1
  f (N)/1 -> Out4/1
  fc (N)/1 -> Out5/1
  tc (Nm)/1 -> Out6/1
  ft (N)/1 -> Out7/1
  tt (Nm)/1 -> Out8/1
  connections:
  q/RConn1 -- p (m)/LConn1
  Conn2/RConn1 -- v (m/s)/LConn1
  Conn3/RConn1 -- a (m/s^2)/LConn1
  Conn4/RConn1 -- f (N)/LConn1
  fc (N)/LConn1 -- Conn5/RConn1
  Conn6/RConn1 -- tc (Nm)/LConn1
  ft (N)/LConn1 -- Conn7/RConn1
  Conn8/RConn1 -- tt (Nm)/LConn1

== matlab function DemonstratorSimscape/Transmission System/Roof Pulley Set/Sheave_02/Bending loss/dr switch ==
  data: w input; dr output; eps_w_sh parameter; dr_wpos input
function dr = fcn(w,eps_w_sh,dr_wpos)

if (w > eps_w_sh)
	dr = dr_wpos;
elseif (w < -eps_w_sh)
	dr = -dr_wpos;
else
	dr = 0;
end

== matlab function DemonstratorSimscape/Transmission System/Anchor and Load/Sheave_03/Bending loss/dr switch ==
  data: w input; dr output; eps_w_sh parameter; dr_wpos input
function dr = fcn(w,eps_w_sh,dr_wpos)

if (w > eps_w_sh)
	dr = dr_wpos;
elseif (w < -eps_w_sh)
	dr = -dr_wpos;
else
	dr = 0;
end

== matlab function DemonstratorSimscape/Transmission System/Anchor and Load/Sheave_05/Bending loss/dr switch ==
  data: w input; dr output; eps_w_sh parameter; dr_wpos input
function dr = fcn(w,eps_w_sh,dr_wpos)

if (w > eps_w_sh)
	dr = dr_wpos;
elseif (w < -eps_w_sh)
	dr = -dr_wpos;
else
	dr = 0;
end

== matlab function DemonstratorSimscape/Transmission System/Roof Pulley Set/Sheave_06/Bending loss/dr switch ==
  data: w input; dr output; eps_w_sh parameter; dr_wpos input
function dr = fcn(w,eps_w_sh,dr_wpos)

if (w > eps_w_sh)
	dr = dr_wpos;
elseif (w < -eps_w_sh)
	dr = -dr_wpos;
else
	dr = 0;
end

== matlab function DemonstratorSimscape/Transmission System/Roof Pulley Set/Sheave_07/Bending loss/dr switch ==
  data: w input; dr output; eps_w_sh parameter; dr_wpos input
function dr = fcn(w,eps_w_sh,dr_wpos)

if (w > eps_w_sh)
	dr = dr_wpos;
elseif (w < -eps_w_sh)
	dr = -dr_wpos;
else
	dr = 0;
end

== matlab function DemonstratorSimscape/Transmission System/Roof Pulley Set/Sheave_01/Bending loss/dr switch ==
  data: w input; dr output; eps_w_sh parameter; dr_wpos input
function dr = fcn(w,eps_w_sh,dr_wpos)

if (w > eps_w_sh)
	dr = dr_wpos;
elseif (w < -eps_w_sh)
	dr = -dr_wpos;
else
	dr = 0;
end
